simulink model "GFLIB_Limit_BAM_FLT"  (Simulink 8.3)
settings: Solver=ode45  StartTime=0.0  StopTime=10.0  RelTol=1e-3
undefined symbols (not defined in the file): fltLowerLim, fltUpperLimit
settings Model: Creator=B17364  LastModifiedBy=B17364
settings OptimizationCC: ExpressionDepthLimit=2147483647
settings DebuggingCC: FcnCallInpInsideContextMsg=UseLocalSettings  StrictBusMsg=Warning

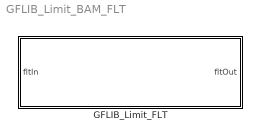
== system GFLIB_Limit_BAM_FLT ==
  GFLIB_Limit_FLT : Subsystem  mask(GFLIB_Limit){fltUpperLimit=fltUpperLimit, fltLowerLim=fltLowerLim}
      mask help: Bit accurate model of the GFLIB_Limit function.
      mask init:
      | pos = get_param(gcb, 'Position');width = pos(3) - pos(1); height = pos(4) - pos(2);tX=width/2;tY=height*0.9;
      mask Display: color('black');port_label('input',1,'fltIn');port_label('output',1,'fltOut');color('black');disp('GFLIB_Limit_FLT');color('blue');text(tX,tY, 'BAM', 'horizontalAlignment', 'center');

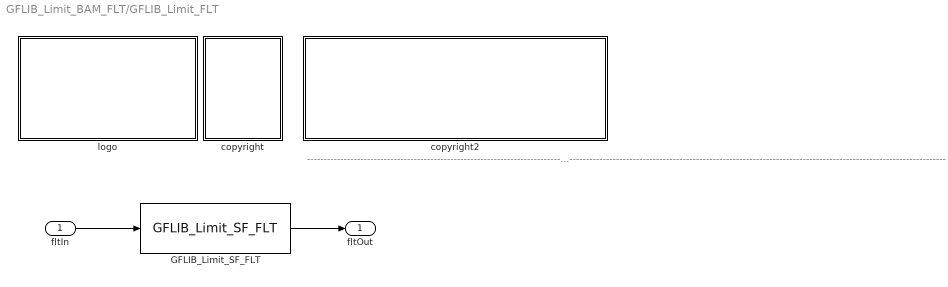
== system GFLIB_Limit_BAM_FLT/GFLIB_Limit_FLT ==
  note: ---------------------------------------------------------------------------------------------------------------------------------------------------------------------------------------------------
  fltIn : Inport
  GFLIB_Limit_SF_FLT : S-Function  FunctionName=GFLIB_Limit_SF_FLT  Parameters=fltUpperLimit,fltLowerLim  EnableBusSupport=off
  copyright : Subsystem
      mask Display:
      | text(10,90,'FILE:');text(10,75,'DESRIPTION:')
      | text(10,60,'COPYRIGHT:')
      | text(10,45,'VERSION:')
      | text(10,30,'DATE:')
      | text(10,15,'AUTHOR:')
  copyright2 : Subsystem
      mask Display:
      | text(10,90,'GFLIB_Limit_BAM_FLT.mdl');text(10,75,'Limit function');text(10,60,'Freescale')
      | text(10,45,'0.1');text(10,30,'03-Jul-2011');text(10,15,'');
  logo : Subsystem
      mask Display: image(imread('logo.jpg'))
  fltOut : Outport
  wires:
  fltIn/1 -> GFLIB_Limit_SF_FLT/1
  GFLIB_Limit_SF_FLT/1 -> fltOut/1

== system GFLIB_Limit_BAM_FLT/GFLIB_Limit_FLT/copyright ==

== system GFLIB_Limit_BAM_FLT/GFLIB_Limit_FLT/copyright2 ==

== system GFLIB_Limit_BAM_FLT/GFLIB_Limit_FLT/logo ==
